simulink model "button_increase_decrease_click"  (R2019b)
settings: Solver=FixedStepAuto  StartTime=0.0  StopTime=inf  FixedStep=1  RelTol=1e-3
settings Model: Creator=ONLY-GOD  LastModifiedBy=ONLY-GOD

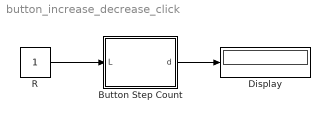
== system button_increase_decrease_click ==
  Button Step Count : MATLAB Function  TreatAsAtomicUnit=on
  Display : Display
  R : Constant
  wires:
  R/1 -> Button Step Count/1(L)
  Button Step Count/1(d) -> Display/1

== matlab function button_increase_decrease_click/Button Step Count ==
  data: d output; L input
function d = fcn(L)
persistent c
if isempty(c) 
    c = 0;end
if L > 0
    d=c+1;
    c = d;
else
    d=c;
end
